simulink model "overview_model"  (R2017b)
settings: Solver=VariableStepAuto  StartTime=0.0  StopTime=10.0  RelTol=1e-3
settings Model: Creator=Joe  LastModifiedBy=Joe

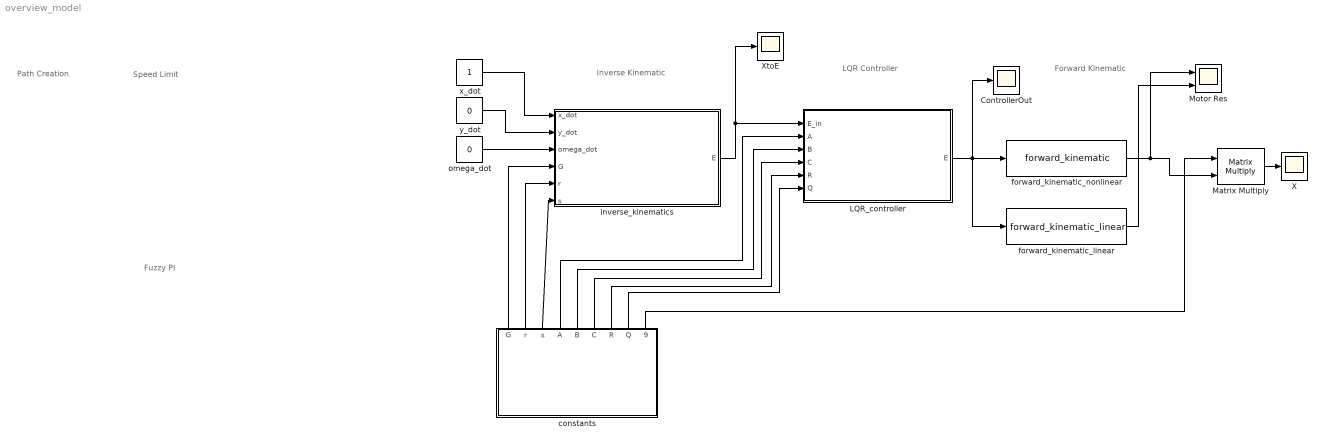
== system overview_model ==
  note: Forward Kinematic
  note: LQR Controller
  note: Inverse Kinematic
  note: Fuzzy PI
  note: Speed Limit
  note: Path Creation
  ControllerOut : Scope
  LQR_controller : MATLAB Function  TreatAsAtomicUnit=on
  Matrix Multiply : Product  Multiplication=Matrix(*)
  Motor Res : Scope  NumInputPorts=2
  X : Scope
  XtoE : Scope
  constants : MATLAB Function  TreatAsAtomicUnit=on
  forward_kinematic_linear : M-S-Function  FunctionName=forward_kinematic_linear
  forward_kinematic_nonlinear : M-S-Function  FunctionName=forward_kinematic
  inverse_kinematics : MATLAB Function  TreatAsAtomicUnit=on
  omega_dot : Constant  Value=0
  x_dot : Constant
  y_dot : Constant  Value=0
  wires:
  inverse_kinematics/1(E) -> LQR_controller/1(E_in), XtoE/1
  constants/4(A) -> LQR_controller/2(A)
  constants/5(B) -> LQR_controller/3(B)
  constants/6(C) -> LQR_controller/4(C)
  constants/7(R) -> LQR_controller/5(R)
  constants/8(Q) -> LQR_controller/6(Q)
  omega_dot/1 -> inverse_kinematics/3(omega_dot)
  y_dot/1 -> inverse_kinematics/2(y_dot)
  x_dot/1 -> inverse_kinematics/1(x_dot)
  constants/1(G) -> inverse_kinematics/4(G)
  constants/2(r) -> inverse_kinematics/5(r)
  constants/3(s) -> inverse_kinematics/6(s)
  LQR_controller/1(E) -> forward_kinematic_linear/1, ControllerOut/1, forward_kinematic_nonlinear/1
  Matrix Multiply/1 -> X/1
  constants/9(G_inv_r) -> Matrix Multiply/1
  forward_kinematic_nonlinear/1 -> Motor Res/1, Matrix Multiply/2
  forward_kinematic_linear/1 -> Motor Res/2

== matlab function overview_model/inverse_kinematics ==
  data: x_dot input; y_dot input; omega_dot input; E output; G input; r input; s input
function E  = inverse_kinematics(x_dot, y_dot, omega_dot, G, r, s)
    E = G' * [x_dot;y_dot;omega_dot] ./ r ./(2*pi) ./ s .* 60;
end

== matlab function overview_model/LQR_controller ==
  data: E_in input; E output; A input; B input; C input; R input; Q input
function E = LQR_controller(E_in, A, B, C, R, Q)
    E = E_in;
end

== matlab function overview_model/constants ==
  data: G output; r output; s output; A output; B output; C output; R output; Q output; G_inv_r output
function [G, r, s, A, B, C, R, Q, G_inv_r] = constants()
Rt = 0.978;
k_m = 33.5 * 1000;
EM = 1/285;
J_L = 2.158e-5;
J_m = 1.35e-5;
J = 0.013;
l = 0.0824;
m = 3.678;
n = 4.091;
r = 0.0285;
c_m = 0;
c_L = 0;
s = 1 / EM;

A = zeros(4,4);
B = zeros(4,4);
C = zeros(4,4);
R = zeros(4,4);
Q = zeros(4,4);

theta = [0, pi/2, pi, 3*pi/2];
G = [-sin(theta(1)), -sin(theta(2)), -sin(theta(3)), -sin(theta(4));
      cos(theta(1)),  cos(theta(2)),  cos(theta(3)),  cos(theta(4));
                  l,              l,              l,              l];
                  
G_inv_r = pinv(G')*r*2*pi;
end
